simulink model "Demo"  (R2021b)
settings: configuration reference "config_demo" (kept outside this file)
settings Model: Creator=julie  LastModifiedBy=julie
settings ConfigSetRef: SourceName=config_demo  SourceLocation=Base Workspace

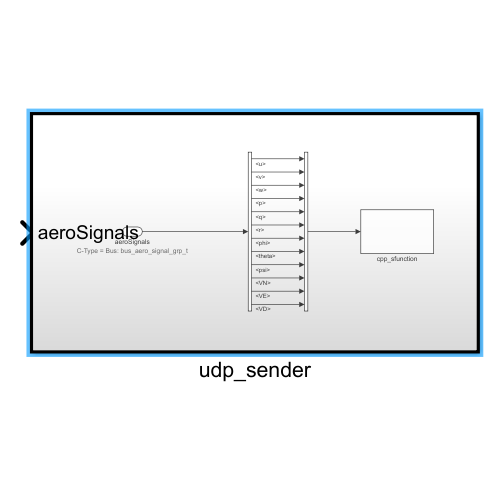
[thumbnail: Simulink's stored preview of the top-level diagram]
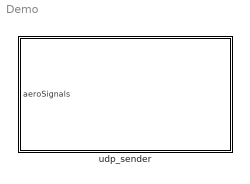
== system Demo ==
  udp_sender : Subsystem  TreatAsAtomicUnit=on

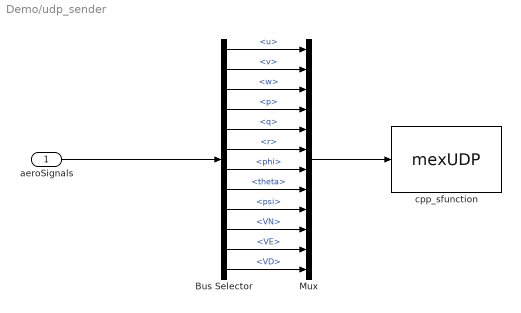
== system Demo/udp_sender ==
  aeroSignals : Inport  OutDataTypeStr=Bus: bus_aero_signal_grp_t
      settings: AttributesFormatString=C-Type = %<OutDataTypeStr>
  Bus Selector : BusSelector  OutputSignals=u,v,w,p,q,r,phi,theta,psi,VN,VE,VD
  Mux : Mux  Inputs=12
  cpp_sfunction : S-Function  FunctionName=mexUDP  SFunctionDeploymentMode=off  EnableBusSupport=off
  wires:
  aeroSignals/1 -> Bus Selector/1
  Bus Selector/1 -> Mux/1  "<u>"
  Bus Selector/2 -> Mux/2  "<v>"
  Bus Selector/3 -> Mux/3  "<w>"
  Bus Selector/4 -> Mux/4  "<p>"
  Bus Selector/5 -> Mux/5  "<q>"
  Bus Selector/6 -> Mux/6  "<r>"
  Bus Selector/7 -> Mux/7  "<phi>"
  Bus Selector/8 -> Mux/8  "<theta>"
  Bus Selector/9 -> Mux/9  "<psi>"
  Bus Selector/10 -> Mux/10  "<VN>"
  Bus Selector/11 -> Mux/11  "<VE>"
  Bus Selector/12 -> Mux/12  "<VD>"
  Mux/1 -> cpp_sfunction/1
